simulink model "pi_controller"  (R2017a)
settings: Solver=FixedStepAuto  StartTime=0.0  StopTime=inf  RelTol=1e-3  EnableMultiTasking=on
libraries: raspberrypilib x1
settings Model: SimulationMode=external  Creator=Vincent  LastModifiedBy=Vincent
settings SolverCC: PositivePriorityOrder=on
settings OptimizationCC: PassReuseOutputArgsThreshold=0  MaxStackSize=64
settings DebuggingCC: ParameterTunabilityLossMsg=error
settings HardwareCC: ProdBitPerPointer=32  ProdBitPerSizeT=32  ProdBitPerPtrDiffT=32  ProdLargestAtomicInteger=Long  ProdLargestAtomicFloat=Double  ProdWordSize=32  ProdHWDeviceType=ARM Compatible->ARM Cortex
settings SFSimCC: MATLABDynamicMemAlloc=off
settings RTWCC: SystemTargetFile=ert.tlc  HardwareBoard=Raspberry Pi  TLCOptions="-aInlineSetEventsForThisBaseRateFcn=TLC_FALSE -aSuppressMultiTaskScheduler=TLC_FALSE  -aRateBasedStepFcn=0"  TemplateMakefile=ert_default_tmf  Description=Embedded Coder  GenerateReport=on  Toolchain=GNU GCC Raspberry Pi  LaunchReport=on
settings CodeAppCC: ForceParamTrailComments=on  OperatorAnnotations=on  MATLABSourceComments=on
settings ERTTargetCC: ERTCustomFileBanners=off  SupportContinuousTime=on  SupportNonInlinedSFcns=on  RemoveResetFunc=off  SupportVariableSizeSignals=on  ModelStepFunctionPrototypeControlCompliant=off

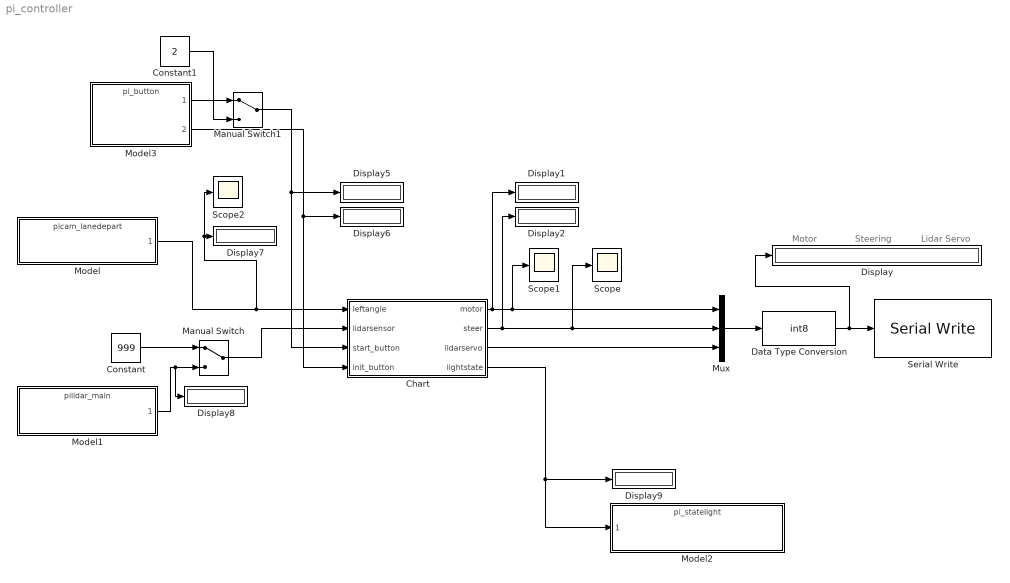
== system pi_controller ==
  note: Motor
  note: Steering
  note: Lidar Servo
  Chart : Stateflow chart  TreatAsAtomicUnit=on
  Constant : Constant  Value=999
  Constant1 : Constant  Value=2
  Data Type Conversion : DataTypeConversion  OutDataTypeStr=int8
  Display{,1..2,5..9} (8 alike) : Display
  Manual Switch : ManualSwitch
  Manual Switch1 : ManualSwitch
  Model : ModelReference  ModelNameDialog=picam_lanedepart.slx  SimulationMode=Normal  ModelReferenceVersion=1.12
  Model1 : ModelReference  ModelNameDialog=pilidar_main.slx  SimulationMode=Normal  ModelReferenceVersion=1.10
  Model2 : ModelReference  ModelNameDialog=pi_statelight.slx  SimulationMode=Normal  ModelReferenceVersion=1.6
  Model3 : ModelReference  ModelNameDialog=pi_button  SimulationMode=Normal  ModelReferenceVersion=1.9
  Mux : Mux  Inputs=3
  Scope : Scope
  Scope1 : Scope
  Scope2 : Scope
  Serial Write : raspberrypilib/Serial Write  board=Pi 3 Model B  SCIModule_=/dev/ttyS0  Baudrate_=9600  Parity=None  StopBits_=1  HardwareFlowControl=None  ByteOrder=LittleEndian  OutputStatus=off  blockPlatform=RaspberryPi
      settings: SourceProductName=Simulink Support Package for Raspberry Pi Hardware  SourceProductBaseCode=RASPPI
  wires:
  Manual Switch/1 -> Chart/2(lidarsensor)
  Constant/1 -> Manual Switch/1
  Model1/1 -> Display8/1, Manual Switch/2
  Chart/4(lightstate) -> Display9/1, Model2/1
  Model3/2 -> Display6/1, Chart/4(init_button)
  Chart/2(steer) -> Display2/1, Mux/2, Scope/1
  Chart/3(lidarservo) -> Mux/3
  Chart/1(motor) -> Mux/1, Scope1/1, Display1/1
  Data Type Conversion/1 -> Display/1, Serial Write/1
  Mux/1 -> Data Type Conversion/1
  Manual Switch1/1 -> Display5/1, Chart/3(start_button)
  Model3/1 -> Manual Switch1/1
  Constant1/1 -> Manual Switch1/2
  Model/1 -> Scope2/1, Display7/1, Chart/1(leftangle)

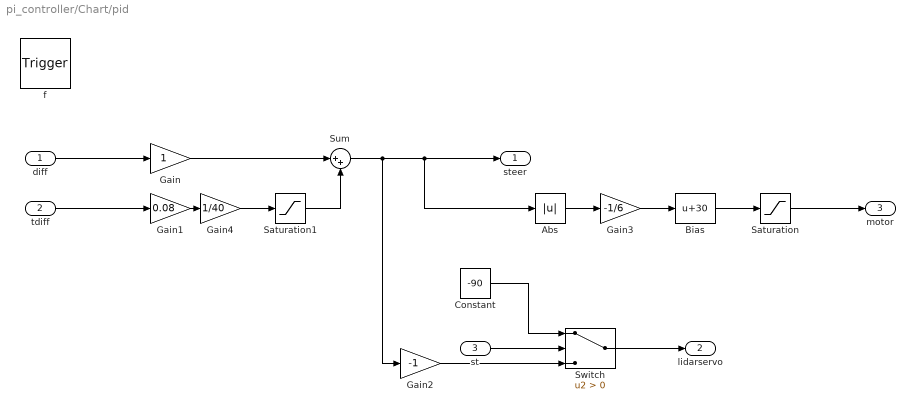
== system pi_controller/Chart/pid ==
  diff : Inport  OutDataTypeStr=double  PortDimensions=1
  tdiff : Inport  Port=2  OutDataTypeStr=double  PortDimensions=1
  st : Inport  Port=3  OutDataTypeStr=double  PortDimensions=1
  f : TriggerPort  TriggerType=function-call  VariantControl=Variant
      settings: CopyFcn=Stateflow.SLINSF.SimulinkMan.removeBlockPreDeleteFcn  PreDeleteFcn=Stateflow.SLINSF.SimulinkMan.unsafePredeleteFcn
  Abs : Abs
  Bias : Bias  Bias=30
  Constant : Constant  Value=-90
  Gain : Gain
  Gain1 : Gain  Gain=0.08
  Gain2 : Gain  Gain=-1
  Gain3 : Gain  Gain=-1/6
  Gain4 : Gain  Gain=1/40
  Saturation : Saturate  UpperLimit=30  LowerLimit=15
  Saturation1 : Saturate  UpperLimit=30  LowerLimit=0
  Sum : Sum  Inputs=|++
  Switch : Switch  Criteria=u2 > Threshold
  steer : Outport
  lidarservo : Outport  Port=2
  motor : Outport  Port=3
  wires:
  tdiff/1 -> Gain1/1
  Gain/1 -> Sum/1
  Gain1/1 -> Gain4/1
  Gain3/1 -> Bias/1
  Saturation/1 -> motor/1
  Bias/1 -> Saturation/1
  Abs/1 -> Gain3/1
  Sum/1 -> Gain2/1, Abs/1, steer/1
  Gain2/1 -> Switch/3
  Switch/1 -> lidarservo/1
  Constant/1 -> Switch/1
  st/1 -> Switch/2
  Gain4/1 -> Saturation1/1
  Saturation1/1 -> Sum/2
  diff/1 -> Gain/1

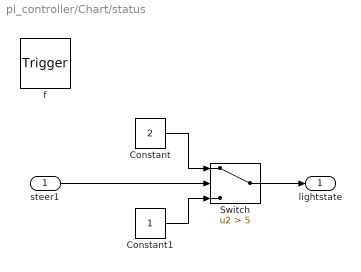
== system pi_controller/Chart/status ==
  steer1 : Inport  OutDataTypeStr=double  PortDimensions=1
  f : TriggerPort  TriggerType=function-call  VariantControl=Variant
      settings: CopyFcn=Stateflow.SLINSF.SimulinkMan.removeBlockPreDeleteFcn  PreDeleteFcn=Stateflow.SLINSF.SimulinkMan.unsafePredeleteFcn
  Constant : Constant  Value=2
  Constant1 : Constant
  Switch : Switch  Criteria=u2 > Threshold  Threshold=5
  lightstate : Outport
  wires:
  steer1/1 -> Switch/2
  Constant/1 -> Switch/1
  Constant1/1 -> Switch/3
  Switch/1 -> lightstate/1

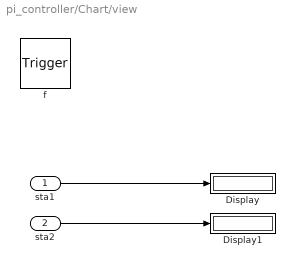
== system pi_controller/Chart/view ==
  sta1 : Inport  OutDataTypeStr=double  PortDimensions=1
  sta2 : Inport  Port=2  OutDataTypeStr=double  PortDimensions=1
  f : TriggerPort  TriggerType=function-call  VariantControl=Variant
      settings: CopyFcn=Stateflow.SLINSF.SimulinkMan.removeBlockPreDeleteFcn  PreDeleteFcn=Stateflow.SLINSF.SimulinkMan.unsafePredeleteFcn
  Display : Display
  Display1 : Display
  wires:
  sta1/1 -> Display/1
  sta2/1 -> Display1/1

== stateflow chart pi_controller/Chart ==
  settings: updateMethod=DISCRETE  sampleTime=1/40
  state pre_start
    entry:
    st = 999;
  state init
    entry:
    time = 0;
    lightstate = 2;
    cangle = leftangle
    st = 0;
    during:
    time = time + 1/40
  state start
    during:
    lightstate = 0;
  state start_2
    entry:
    cangle = leftangle;
  state start_1
  state [steer, lidarservo, motor] = pid(diff,tdiff,st) [function]
  state steady
    entry:
    diff = 0; tdiff = 0;
    time = 0;
    lightstate = 0;
    motor = 50; steer = 0; lidarservo = 0;
    during:
    view(cangle,leftangle)
    st = 0;
    saveangle = leftangle;
    diff = leftangle - cangle; tdiff = tdiff + diff;
    [steer, lidarservo, motor] = pid(diff, tdiff, st);
    lightstate = status(steer);
  state evade_obstacle
    entry:
    time = 0;
    during:
    motor = 20; steer = 45; lidarservo = -45;
    time = time + 1/40;
    lightstate = 3;
  state lightstate = status(steer1) [function]
  state view(sta1, sta2) [function]
  state wait_to_return
    during:
    st = 1;
    saveangle = leftangle;
    diff = leftangle - cangle; tdiff = tdiff + diff;
    [steer, lidarservo, motor] = pid(diff, tdiff, st);
    lightstate = status(steer);
  state wait_to_return1
    entry:
    time = 0;
    during:
    time = time + 1/40;
  state return_to_lane
    entry:
    time = 0;
    during:
    motor = 20; steer = -45; lidarservo = 45;
    time = time + 1/40;
    lightstate = 3;
  (default) -> pre_start
  pre_start -> start
  return_to_lane -> start [order 2] : [start_button == 1]
  init -> start : [time >= 0.5]
  wait_to_return -> start [order 2] : [start_button == 1]
  evade_obstacle -> start [order 2] : [start_button == 1]
  start -> init [order 3] : [init_button == 1]
  steady -> start [order 2] : [start_button == 1]
  start -> start_2 [order 1] : [start_button == 2]
  start_1 -> start [order 2]
  start -> start_1 [order 2] : [start_button == 1]
  start_1 -> steady [order 1] : [st == 0]
  start_2 -> steady
  steady -> evade_obstacle [order 1] : [lidarsensor < 40]
  evade_obstacle -> wait_to_return [order 1] : [time >= 0.8]
  wait_to_return -> wait_to_return1 [order 1] : [lidarsensor >= 40]
  wait_to_return1 -> wait_to_return [order 1] : [lidarsensor < 20]
  wait_to_return1 -> return_to_lane [order 2] : [time >= 1]
  return_to_lane -> steady [order 1] : [time >= 0.8]
  data: diff function_input double size=1; steer function_output; lidarservo function_output; tdiff function_input double size=1; motor function_output; st function_input double size=1; steer1 function_input double size=1; lightstate function_output; sta1 function_input double size=1; sta2 function_input double size=1; leftangle input size=1; lidarsensor input size=1; motor output size=1; steer output size=1; lidarservo output size=1; lightstate output size=1; cangle local size=1; diff local size=1; tdiff local size=1; time local size=1; start_button input size=1; saveangle local size=1; st local size=1; init_button input size=1; st1 local size=1; st2 local size=1
